simulink model "robot"  (R2021a)
settings: Solver=ode23tb  StartTime=0.0  StopTime=10.0  RelTol=P_rt
PreLoadFcn:
  | robot_data;
InitFcn:
  | robot_data;
values from neighbouring files (symbols this model uses):
  P_g = 9.81    [robot_data.m]
  P_l1 = 0.8    [robot_data.m]
  P_l2 = 0.7    [robot_data.m]
  P_m1 = 10    [robot_data.m]
  P_m2 = 10    [robot_data.m]
  u_1s = (P_m1+P_m2)*P_g*P_l1*sin(x_0(1)) + u_2s    [robot_data.m]
  u_2s = P_m2*P_g*P_l2*sin(x_0(2))    [robot_data.m]
  x_0 = [pi; pi/2; 0; 0]    [robot_data.m]
settings Model: EnablePacing=on  Creator=matti  LastModifiedBy=matti

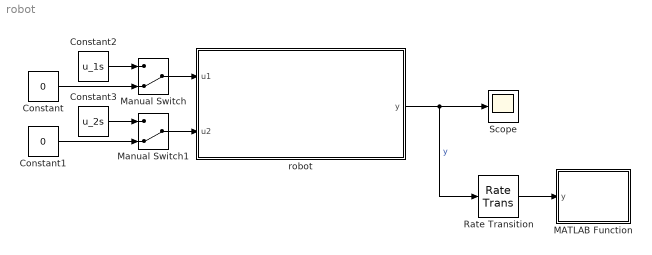
== system robot ==
  Constant : Constant  Value=0
  Constant1 : Constant  Value=0
  Constant2 : Constant  Value=u_1s
  Constant3 : Constant  Value=u_2s
  MATLAB Function : MATLAB Function  TreatAsAtomicUnit=on
  Manual Switch : ManualSwitch  CurrentSetting=0
  Manual Switch1 : ManualSwitch  CurrentSetting=0
  Rate Transition : RateTransition  OutPortSampleTime=P_Ts
  Scope : Scope
  robot : Subsystem
  wires:
  robot/1(y) -> Rate Transition/1, Scope/1  "y"
  Rate Transition/1 -> MATLAB Function/1(y)
  Manual Switch/1 -> robot/1(u1)
  Manual Switch1/1 -> robot/2(u2)
  Constant1/1 -> Manual Switch1/2
  Constant/1 -> Manual Switch/2
  Constant2/1 -> Manual Switch/1
  Constant3/1 -> Manual Switch1/1

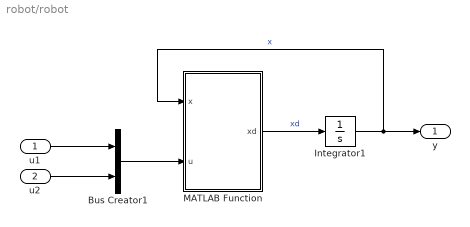
== system robot/robot ==
  u1 : Inport
  u2 : Inport  Port=2
  Bus Creator1 : BusCreator  Inputs=2
  Integrator1 : Integrator  InitialCondition=x_0
  MATLAB Function : MATLAB Function  TreatAsAtomicUnit=on
  y : Outport
  wires:
  MATLAB Function/1(xd) -> Integrator1/1  "xd"
  u1/1 -> Bus Creator1/1
  u2/1 -> Bus Creator1/2
  Bus Creator1/1 -> MATLAB Function/2(u)
  Integrator1/1 -> y/1, MATLAB Function/1(x)  "x"

== matlab function robot/MATLAB Function ==
  data: y input; P_l1 parameter; P_l2 parameter
%% Animation function
function robot_display(y, P_l1, P_l2)
% Animation of the robot with the lower and upper arm as well as 
% the shoulder, elbow and hand
% Input     Type        Description
% y         4x1 double  simulation output
% Parameter Type        Description
% P_l1      1x1 double  upper arm length [ m ]
% P_l2      1x1 double  lower arm length [ m ]
coder.extrinsic('patch');
persistent upperarm;
persistent lowerarm;
persistent shoulder;
persistent elbow;
persistent hand;
%% Parameter and precalculation
width = 0.05;           % width of both arms [m]
radius = 0.05;          % radius of joints [m]
cp1 = cos(y(1));        % cosinus of phi1
sp1 = sin(y(1));        % sinus of phi1
cp2 = cos(y(2));        % cosinus of phi2
sp2 = sin(y(2));        % sinus of phi2
xcu = width/2*cp1;      % corner distance of upper arm in x direction [m]
ycu = width/2*sp1;      % corner distance of upper arm in y direction [m]
xcl = width/2*cp2;      % corner distance of lower arm in x direction [m]
ycl = width/2*sp2;      % corner distance of lower arm in y direction [m]
x1 = sp1*P_l1;          % x-position of the elbow [m]
y1 = -cp1*P_l1;         % y-position of the elbow [m]
x2 = x1+sp2*P_l2;       % x-position of the hand [m]
y2 = y1-cp2*P_l2;       % y-position of the hand [m]

%% Rectangle definition of upper and lower arm
upperarmx = [-xcu; xcu; x1+xcu; x1-xcu];
upperarmy = [-ycu; ycu; y1+ycu; y1-ycu];
lowerarmx = [x1-xcl; x1+xcl; x2+xcl; x2-xcl];
lowerarmy = [y1-ycl; y1+ycl; y2+ycl; y2-ycl];

%% Circle (octagon) definition of shoulder, elbow and hand
% modify for polygon with more corners
% alpha = 0:pi/4:7/4*pi;
% a = transpose(alpha);
% shoulderx = cos(a).*radius;
% shouldery = sin(a).*radius;
% octagon
r45 = radius/sqrt(2);   % value of x, y at 45° [m]
shoulderx = [radius; r45; 0; -r45; -radius; -r45; 0; r45];
shouldery = [0; r45; radius; r45; 0; -r45; -radius; -r45];
elbowx = shoulderx+x1;
elbowy = shouldery+y1;
handx = shoulderx+x2;
handy = shouldery+y2;

%% Animation
if isempty(lowerarm)% && isempty(upperarm) && isempty(shoulder) && isempty(elbow) && isempty(hand)
    figure(1);
    clf;
    title('Animation des Zwei-Gelenk-Roboters');
    axis([-2 2 -2 2]);
    axis equal;
    axis manual;
    grid on;
    hold on;
    upperarm = patch(upperarmx, upperarmy, [0;0;0;0],...
        'FaceColor', 'r', 'EdgeColor', 'r');
    lowerarm = patch(lowerarmx, lowerarmy, [0;0;0;0],...
        'FaceColor', 'r', 'EdgeColor', 'r');
    shoulder = patch(shoulderx, shouldery, zeros(8,1),...
        'FaceColor', 'k', 'EdgeColor', 'k');
    elbow = patch(elbowx, elbowy, zeros(8,1),...
        'FaceColor', 'k', 'EdgeColor', 'k');
    hand = patch(handx, handy, zeros(8,1),...
        'FaceColor', 'k', 'EdgeColor', 'k');

end

set(upperarm, 'XData', upperarmx);
set(upperarm, 'YData', upperarmy);
set(upperarm, 'FaceColor', 'r');
set(lowerarm, 'XData', lowerarmx);
set(lowerarm, 'YData', lowerarmy);
set(lowerarm, 'FaceColor', 'r');
set(shoulder, 'XData', shoulderx);
set(shoulder, 'YData', shouldery);
set(shoulder, 'FaceColor', 'k');
set(elbow, 'XData', elbowx);
set(elbow, 'YData', elbowy);
set(elbow, 'FaceColor', 'k');
set(hand, 'XData', handx);
set(hand, 'YData', handy);
set(hand, 'FaceColor', 'k');

end

== matlab function robot/MATLAB Function ==
  data: x input; xd output; u input; P_m1 parameter; P_m2 parameter; P_l1 parameter; P_l2 parameter; P_g parameter
%% Right hand side of differential equation system
function xd  = rhs_robot(x,u,P_m1, P_m2, P_l1, P_l2, P_g)
% Input     Type        Description
% x         4x1 double  states
% u         2x1 double  inputs
% Parameter Type        Description
% P_m1      1x1 double  elbow motor mass [ kg ]
% P_m2      1x1 double  robot load mass [ kg ]
% P_l1      1x1 double  upper arm length [ m ]
% P_l2      1x1 double  lower arm length [ m ]
% P_g       1x1 double  gravity [ m/s^2 ]
% Output    Type        Description
% xd        4x1 double  derivative of states

% Precalculation
cph = cos(x(1)-x(2));
sph = sin(x(1)-x(2));

% Inverse of mass matrix M
Minv = [P_m2*P_l2*P_l2, -P_m2*P_l1*P_l2*cph;...
    -P_m2*P_l1*P_l2*cph,(P_m1+P_m2)*P_l1*P_l1]...
    /(P_l1*P_l1 * P_l2*P_l2 * (P_m1*P_m2 + P_m2*P_m2 * (1-cph*cph)));
% rest of ride hand side
F = ([P_m2*P_l1*P_l2*sph*x(4)*x(4);...
    -P_m2*P_l1*P_l2*sph*x(3)*x(3)]-...
    [(P_m1+P_m2)*P_g*P_l1*sin(x(1));P_m2*P_g*P_l2*sin(x(2))]+...
    [u(1)-u(2);u(2)]);
% Differential equation of xd3 and xd4
xd34 = Minv * F;

xd = [x(3);x(4);xd34];
